simulink model "Adaptive controller"  (R2023b)
settings: Solver=VariableStepAuto  StartTime=0.0  StopTime=100  RelTol=1e-3
InitFcn:
  | clear
  | 
  | % % ---prof params---
  | % b0= 20;
  | % a1= 9;
  | % a0= 20;
  | %
  | % am1= 5;
  | % am0= 6;
  | 
  | % % ---My params ---
  | b0= 3;
  | a1= 3; % previously 3
  | a0= -1; % previously 1
  | 
  | am1= 2;
  | am0= 1;
  | 
  | b0_bar=0.01;
  | gamma0=3000;
  | lambda=1;
  | 
  | d1 = 1;
  | d2 = 3;
  | d3 = 5;
  | 
  | umin=0;
  | umax=2;
settings Model: Creator=Admin  LastModifiedBy=Admin

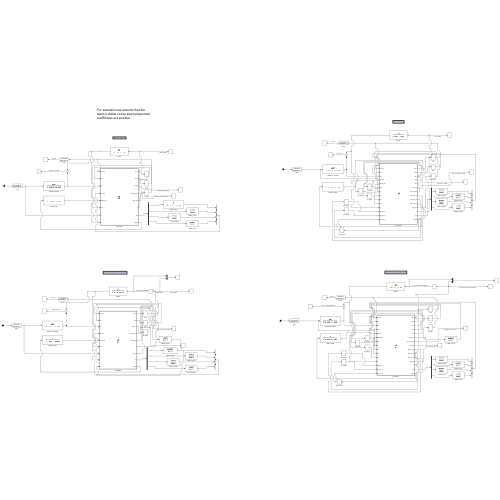
[thumbnail: Simulink's stored preview of the top-level diagram]
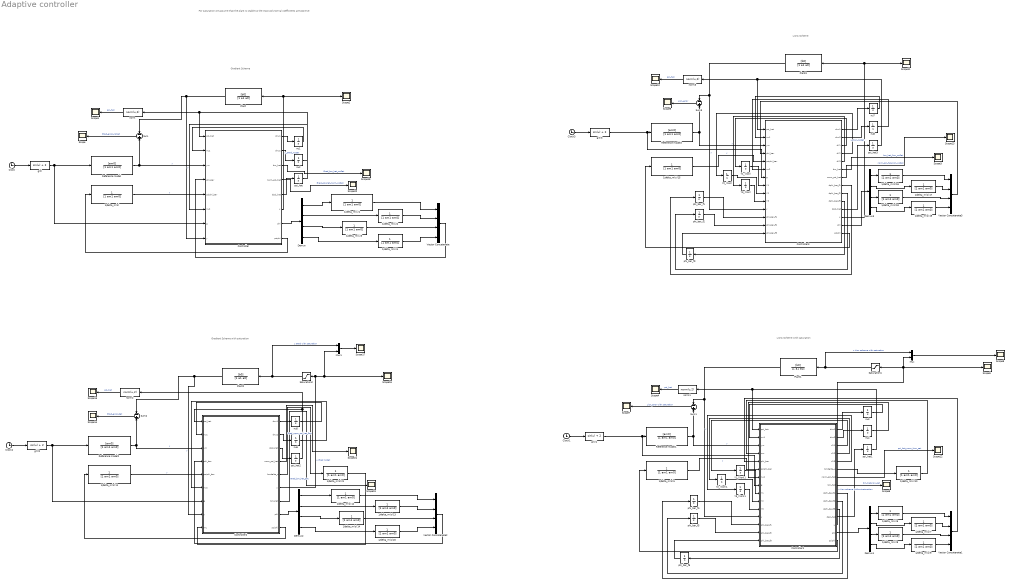
== system Adaptive controller ==
  note: For saturation we assume that the plant is stable so the input polynomial coefficients are positive
  note: Gradient Scheme
  note: Lions Scheme
  note: Lions Scheme with saturation
  note: Gradient Scheme with saturation
  1/delta_m(s){,1..21} (22 alike) : TransferFcn  Denominator=[1 am1 am0]  ParameterTunability=Optimized
  Clock{,1..3} (4 alike) : Clock
  Controller : MATLAB Function  TreatAsAtomicUnit=on
  Controller1 : MATLAB Function  TreatAsAtomicUnit=on
  Controller2 : MATLAB Function  TreatAsAtomicUnit=on
  Controller3 : MATLAB Function  TreatAsAtomicUnit=on
  Demux{,1..3} (4 alike) : Demux
  Mux : Mux  Inputs=2
  Mux1 : Mux  Inputs=2
  Plant{,1..3} (4 alike) : TransferFcn  Numerator=[b0]  Denominator=[1 a1 a0]
  Reference model{,1..3} (4 alike) : TransferFcn  Numerator=[am0]  Denominator=[1 am1 am0]  ParameterTunability=Optimized
  Saturation1 : Saturate  UpperLimit=umax  LowerLimit=umin
  Saturation2 : Saturate  UpperLimit=umax  LowerLimit=umin
  Scope{,1..21} (22 alike) : Scope
  Sum{,1..3} (4 alike) : Sum  Inputs=-+
  Vector Concatenate{,1..3} (4 alike) : Concatenate  NumInputs=4
  Y1_(lion) : Integrator  InitialCondition=[0]
  Y1_(lion)1 : Integrator  InitialCondition=[0]
  Y2_(lion) : Integrator  InitialCondition=[0]
  Y2_(lion)1 : Integrator  InitialCondition=[0]
  Y3_(lion) : Integrator  InitialCondition=[0]
  Y3_(lion)1 : Integrator  InitialCondition=[0]
  g(t){,1..3} (4 alike) : MATLABFcn  MATLABFcn=sin(u) + 2
  norm{,1..3} (4 alike) : MATLABFcn  MATLABFcn=norm(u,2)
  nu{1..8} (8 alike) : Integrator
  phi_bar_f{1..6} (6 alike) : Integrator  InitialCondition=zeros(4,1)
  psi_hat{,1..3} (4 alike) : Integrator  InitialCondition=[0;0;0;1]
  wires:
  1/delta_m(s)1/1 -> Vector Concatenate/1
  Demux/4 -> 1/delta_m(s)4/1
  Demux/1 -> 1/delta_m(s)1/1
  1/delta_m(s)3/1 -> Vector Concatenate/3
  Controller/6(u) -> Scope2/1, Plant/1  "u_Grad_noSat"
  Controller/8(psiphi) -> 1/delta_m(s)/1
  1/delta_m(s)/1 -> Controller/5(psiphi_bar)  "y"
  Plant/1 -> Controller/8(y), Sum/1  "y"
  Controller/2(dnu2) -> nu2/1
  Clock/1 -> g(t)/1
  g(t)/1 -> Controller/7(g), Reference model/1
  Controller/7(phi) -> Demux/1
  Demux/2 -> 1/delta_m(s)2/1
  Reference model/1 -> Controller/3(ym), Sum/2  "y"
  nu1/1 -> Controller/2(nu1)
  Controller/5(dpsi_hat) -> psi_hat/1
  nu2/1 -> Controller/6(nu2)
  psi_hat/1 -> norm/1, Controller/1(psi_hat)
  1/delta_m(s)4/1 -> Vector Concatenate/4
  norm/1 -> Scope1/1  "psi_hat"
  Controller/1(dnu1) -> nu1/1
  Sum/1 -> Scope/1  "Grad_error_noSat"
  Vector Concatenate/1 -> Controller/4(phi_bar)
  Demux/3 -> 1/delta_m(s)3/1
  1/delta_m(s)2/1 -> Vector Concatenate/2
  norm3/1 -> Scope10/1  "psi_hat"
  Vector Concatenate3/1 -> Controller3/4(phi_bar)
  1/delta_m(s)19/1 -> Vector Concatenate3/4
  g(t)3/1 -> Controller3/7(g), Reference model3/1
  1/delta_m(s)17/1 -> Vector Concatenate3/2
  Controller3/12(u) -> Plant3/1, Scope11/1  "u_lion_noSat"
  nu7/1 -> Controller3/2(nu1)
  Controller3/8(dphi_bar_f1) -> phi_bar_f1/1
  Controller3/9(dphi_bar_f2) -> phi_bar_f2/1
  Sum3/1 -> Scope9/1  "Lion_error"
  Demux3/4 -> 1/delta_m(s)19/1
  phi_bar_f3/1 -> Controller3/14(phi_bar_f3)
  1/delta_m(s)18/1 -> Vector Concatenate3/3
  nu8/1 -> Controller3/6(nu2)
  Reference model3/1 -> Sum3/2, Controller3/3(ym)  "y"
  1/delta_m(s)15/1 -> Controller3/5(psiphi_bar)  "y"
  phi_bar_f2/1 -> Controller3/13(phi_bar_f2)
  Y1_(lion)/1 -> Controller3/8(Y1)
  Demux3/2 -> 1/delta_m(s)17/1
  phi_bar_f1/1 -> Controller3/12(phi_bar_f1)
  Controller3/3(dY1) -> Y1_(lion)/1
  Plant3/1 -> Controller3/11(y), Sum3/1  "y"
  Controller3/4(dY2) -> Y2_(lion)/1
  psi_hat3/1 -> Controller3/1(psi_hat), norm3/1
  Y3_(lion)/1 -> Controller3/10(Y3)
  Controller3/5(dY3) -> Y3_(lion)/1
  Demux3/1 -> 1/delta_m(s)16/1
  Y2_(lion)/1 -> Controller3/9(Y2)
  Controller3/1(dnu1) -> nu7/1
  Demux3/3 -> 1/delta_m(s)18/1
  Controller3/10(dphi_bar_f3) -> phi_bar_f3/1
  Clock3/1 -> g(t)3/1
  Controller3/11(dpsi_hat) -> psi_hat3/1
  Controller3/14(psiphi) -> 1/delta_m(s)15/1
  1/delta_m(s)16/1 -> Vector Concatenate3/1
  Controller3/13(phi) -> Demux3/1
  Controller3/2(dnu2) -> nu8/1
  Controller3/6(bm_hat) -> Scope3/1  "bm_hat_lion_noSat"
  Saturation1/1 -> Mux/1, Plant1/1  "u Lion scheme with saturation"
  Controller1/8(bm_hat) -> Scope6/1  "bm_hat_lion_sat"
  phi_bar_f4/1 -> Controller1/13(phi_bar_f1)
  Plant1/1 -> Controller1/12(y), Sum1/1  "y"
  Controller1/1(dnu1) -> nu3/1
  Controller1/14(phi) -> Demux1/1
  norm1/1 -> Scope4/1  "psi_hat"
  Controller1/15(psiphi) -> 1/delta_m(s)5/1
  Demux1/4 -> 1/delta_m(s)9/1
  Controller1/2(dnu2) -> nu4/1
  1/delta_m(s)6/1 -> Vector Concatenate1/1
  Controller1/11(dphi_bar_f3) -> phi_bar_f6/1
  Controller1/5(dY3) -> Y3_(lion)1/1
  Clock1/1 -> g(t)1/1
  Demux1/2 -> 1/delta_m(s)7/1
  nu3/1 -> Controller1/2(nu1)
  Reference model1/1 -> Sum1/2, Controller1/3(ym)  "y"
  Controller1/3(dY1) -> Y1_(lion)1/1
  1/delta_m(s)5/1 -> Controller1/6(psiphi_bar)  "y"
  Demux1/1 -> 1/delta_m(s)6/1
  Controller1/13(u) -> Scope5/1, Saturation1/1, Mux/2  "u Lion scheme without saturation"
  Y3_(lion)1/1 -> Controller1/11(Y3)
  Y1_(lion)1/1 -> Controller1/9(Y1)
  Demux1/3 -> 1/delta_m(s)8/1
  Controller1/4(dY2) -> Y2_(lion)1/1
  Controller1/9(dphi_bar_f1) -> phi_bar_f4/1
  nu4/1 -> Controller1/7(nu2)
  1/delta_m(s)9/1 -> Vector Concatenate1/4
  psi_hat1/1 -> Controller1/1(psi_hat), norm1/1
  phi_bar_f5/1 -> Controller1/14(phi_bar_f2)
  phi_bar_f6/1 -> Controller1/15(phi_bar_f3)
  1/delta_m(s)8/1 -> Vector Concatenate1/3
  Sum1/1 -> Scope7/1  "Lion_error with saturation"
  Vector Concatenate1/1 -> Controller1/5(phi_bar)
  Controller1/10(dphi_bar_f2) -> phi_bar_f5/1
  Y2_(lion)1/1 -> Controller1/10(Y2)
  1/delta_m(s)7/1 -> Vector Concatenate1/2
  Controller1/12(dpsi_hat) -> psi_hat1/1
  g(t)1/1 -> Controller1/8(g), Reference model1/1
  Controller1/6(bmdelta_u) -> 1/delta_m(s)10/1
  1/delta_m(s)10/1 -> Controller1/4(mu)
  Mux/1 -> Scope8/1
  Controller1/7(norm_psi_hat) -> Scope12/1  "psi_hat_norm_Lion_sat"
  Controller3/7(norm_psi_hat) -> Scope13/1  "norm_psi_hat_lion_noSat"
  Demux2/4 -> 1/delta_m(s)20/1
  Demux2/1 -> 1/delta_m(s)12/1
  1/delta_m(s)11/1 -> Controller2/5(psiphi_bar)  "y"
  psi_hat2/1 -> norm2/1, Controller2/1(psi_hat)
  nu6/1 -> Controller2/6(nu2)
  g(t)2/1 -> Controller2/7(g), Reference model2/1
  Controller2/6(u) -> Scope16/1, Mux1/2, Saturation2/1  "u Grad noSat"
  nu5/1 -> Controller2/2(nu1)
  1/delta_m(s)14/1 -> Vector Concatenate2/3
  Clock2/1 -> g(t)2/1
  1/delta_m(s)20/1 -> Vector Concatenate2/4
  Controller2/2(dnu2) -> nu6/1
  Sum2/1 -> Scope14/1  "Grad_error_Sat"
  Demux2/3 -> 1/delta_m(s)14/1
  Vector Concatenate2/1 -> Controller2/4(phi_bar)
  Reference model2/1 -> Sum2/2, Controller2/3(ym)  "y"
  Controller2/8(phi) -> Demux2/1
  1/delta_m(s)13/1 -> Vector Concatenate2/2
  Demux2/2 -> 1/delta_m(s)13/1
  Controller2/1(dnu1) -> nu5/1
  Controller2/3(dpsi_hat) -> psi_hat2/1
  Controller2/9(psiphi) -> 1/delta_m(s)11/1
  Plant2/1 -> Controller2/8(y), Sum2/1  "y"
  norm2/1 -> Scope15/1  "psi_hat"
  1/delta_m(s)12/1 -> Vector Concatenate2/1
  Saturation2/1 -> Mux1/1, Plant2/1  "u Grad with saturation"
  Mux1/1 -> Scope17/1
  Controller/3(bm_hat) -> Scope18/1  "Grad_bm_hat_noSat"
  Controller2/7(bm_hat) -> Scope19/1  "Grad_bm_hat_Sat"
  Controller/4(norm_psi_hat) -> Scope20/1  "Grad_psi_hat_norm_noSat"
  Controller2/4(norm_psi_hat) -> Scope21/1  "Grad_norm_psi_hat_Sat"
  Controller2/5(bmdelta_u) -> 1/delta_m(s)21/1
  1/delta_m(s)21/1 -> Controller2/9(mu)

== matlab function Adaptive controller/Controller2 ==
  data: psi_hat input; dnu1 output; nu1 input; ym input; phi_bar input; psiphi_bar input; nu2 input; g input; y input; b0_bar parameter; mu input; dnu2 output; dpsi_hat output; norm_psi_hat output; bmdelta_u output; u output; bm_hat output; phi output; psiphi output; gamma0 parameter; am0 parameter; lambda parameter; umin parameter; umax parameter
function [dnu1, dnu2, dpsi_hat, norm_psi_hat, bmdelta_u, u, bm_hat, phi, psiphi] = fcn(psi_hat, nu1, ym, phi_bar,....
    psiphi_bar, nu2, g, y, b0_bar, mu, gamma0, am0, lambda, umin, umax)


% === Initialize Outputs ===
dnu1 = 0;
dnu2 = 0;
dpsi_hat = zeros(4,1);
u = 0;
psi_hat = psi_hat(:);  
phi_bar = phi_bar(:);
phi = zeros(4,1);
psiphi = 0;
bmdelta_u = 0;

% Extract parameters as COLUMN vector
theta_hat = psi_hat(1:3);   

bm_hat = psi_hat(4);        

% Regressor
omega = [y; nu1; nu2];     

% Tracking error
epsilon = ym - y - mu;

% Augmented error
epsilon_hat = epsilon - (psi_hat' * phi_bar) + psiphi_bar;

% Control law — now dimensionally correct
u = (1 / bm_hat) * (-theta_hat' * omega + am0 * g);

% === Apply Saturation ===
Us = u;
if u <= umin
    Us = umin;
elseif u >= umax
    Us = umax;
end

% === Correction Term ===
bmdelta_u = bm_hat * (u - Us);
 
phi = [-omega; -Us];
psiphi = psi_hat'*phi;
omega_bar = -[phi_bar(1); phi_bar(2); phi_bar(3)];

gamma0=gamma0*eye(4); coord=[0;0;0;1];
 
if bm_hat<b0_bar
    gamma0=gamma0*(eye(4)-coord*coord');
end
 
% Normalize gamma based on regressor energy
denom = 1 + omega_bar' * omega_bar;  
gamma = gamma0 / denom;       

% Final adaptation law
dpsi_hat = gamma * phi_bar * epsilon_hat;

% Derivatives for filters
dnu1 = -lambda*nu1+y;
dnu2 = -lambda*nu2+Us;

% Output psiphi if needed
psiphi = psi_hat' * phi;

% Compute Euclidean norm of psi_hat
norm_psi_hat = norm(psi_hat);  
 
end

== matlab function Adaptive controller/Controller3 ==
  data: psi_hat input; dnu1 output; nu1 input; ym input; phi_bar input; psiphi_bar input; nu2 input; g input; Y1 input; Y2 input; Y3 input; y input; dnu2 output; dY1 output; dY2 output; dY3 output; bm_hat output; norm_psi_hat output; dphi_bar_f1 output; dphi_bar_f2 output; dphi_bar_f3 output; dpsi_hat output; u output; phi output; psiphi output; b0_bar parameter; phi_bar_f1 input; phi_bar_f2 input; phi_bar_f3 input; gamma0 parameter; am0 parameter; lambda parameter; d1 parameter; d2 parameter; d3 parameter
function [dnu1, dnu2, dY1, dY2, dY3,bm_hat, norm_psi_hat, dphi_bar_f1, dphi_bar_f2, dphi_bar_f3, dpsi_hat, u, phi, psiphi] = ...
    fcn(psi_hat, nu1, ym, phi_bar, psiphi_bar, nu2, g, Y1, Y2, Y3, y, b0_bar, ...
        phi_bar_f1, phi_bar_f2, phi_bar_f3, gamma0, am0, lambda, d1, d2, d3)

% === Initialize Outputs ===
dnu1 = 0;
dnu2 = 0;
dY1 = 0;
dY2 = 0;
dY3 = 0;
dphi_bar_f1 = zeros(4,1);
dphi_bar_f2 = zeros(4,1);
dphi_bar_f3 = zeros(4,1);
dpsi_hat = zeros(4,1);
u = 0;
phi = zeros(4,1);
psiphi = 0;

% === Input Handling ===
psi_hat = psi_hat(:);           
phi_bar = phi_bar(:);           
psiphi_bar = psiphi_bar(:);

% Filter states
phi_bar_f1 = phi_bar_f1(:);     
phi_bar_f2 = phi_bar_f2(:);     
phi_bar_f3 = phi_bar_f3(:);     

% === Extract Parameters ===
theta_hat = psi_hat(1:3);       
bm_hat = psi_hat(4);            

% === Regressor ===
omega = [y; nu1; nu2];          

% === Tracking Error ===
epsilon = ym - y;              

% === Augmented Error Estimate ===
y_hat = epsilon + psiphi_bar;   

% === Control Law ===
u = (1 / bm_hat) * (-theta_hat' * omega + am0 * g);

% === Extended Regressor ===
phi = [-omega; -u];             
psiphi = psi_hat' * phi;        

% === Adaptation Gain Normalization ===
omega_bar = -[phi_bar(1); phi_bar(2); phi_bar(3)]; 
denom = 1 + omega_bar' * omega_bar;  
gamma_scalar = gamma0 / denom;
gamma = gamma_scalar * eye(4);       

% === Derivatives of Filtered Signals ===
dY1 = -d1*Y1 + d1*y_hat;
dY2 = -d2*Y2 + d2*y_hat;
dY3 = -d3*Y3 + d3*y_hat;

dphi_bar_f1 = -d1*phi_bar_f1 + d1*phi_bar;
dphi_bar_f2 = -d2*phi_bar_f2 + d2*phi_bar;
dphi_bar_f3 = -d3*phi_bar_f3 + d3*phi_bar;

% === Compute Parametric Error for Each Filter Channel ===
E1 = Y1 - phi_bar_f1' * psi_hat;  
E2 = Y2 - phi_bar_f2' * psi_hat;  
E3 = Y3 - phi_bar_f3' * psi_hat;  

% === Final Adaptation Law ===
TotalUpdate = phi_bar_f1 * E1 + phi_bar_f2 * E2 + phi_bar_f3 * E3;
dpsi_hat = gamma * TotalUpdate;  

% === State Filters Derivatives ===
dnu1 = -lambda * nu1 + y;
dnu2 = -lambda * nu2 + u;

% Compute Euclidean norm of psi_hat
norm_psi_hat = norm(psi_hat);  

% === Output psiphi ===
psiphi = psi_hat' * phi;

end

== matlab function Adaptive controller/Controller1 ==
  data: psi_hat input; dnu1 output; nu1 input; ym input; mu input; phi_bar input; psiphi_bar input; nu2 input; g input; Y1 input; Y2 input; Y3 input; y input; dnu2 output; dY1 output; dY2 output; dY3 output; bmdelta_u output; norm_psi_hat output; bm_hat output; dphi_bar_f1 output; dphi_bar_f2 output; dphi_bar_f3 output; dpsi_hat output; u output; phi output; psiphi output; b0_bar parameter; phi_bar_f1 input; phi_bar_f2 input; phi_bar_f3 input; gamma0 parameter; am0 parameter; lambda parameter; d1 parameter; d2 parameter; d3 parameter; umin parameter; umax parameter
function [dnu1, dnu2, dY1, dY2, dY3, bmdelta_u, norm_psi_hat, bm_hat, dphi_bar_f1, dphi_bar_f2, dphi_bar_f3, dpsi_hat, u, phi, psiphi] = ...
    fcn(psi_hat, nu1, ym, mu, phi_bar, psiphi_bar, nu2, g, Y1, Y2, Y3, y, b0_bar, ...
        phi_bar_f1, phi_bar_f2, phi_bar_f3, gamma0, am0, lambda, d1, d2, d3, umin, umax)

% === Initialize Outputs ===
dnu1 = 0;
dnu2 = 0;
dY1 = 0;
dY2 = 0;
dY3 = 0;
dphi_bar_f1 = zeros(4,1);
dphi_bar_f2 = zeros(4,1);
dphi_bar_f3 = zeros(4,1);
dpsi_hat = zeros(4,1);
u = 0;
phi = zeros(4,1);
psiphi = 0;

% === Input Handling ===
psi_hat = psi_hat(:);           
phi_bar = phi_bar(:);           
psiphi_bar = psiphi_bar(:);

% Filter states
phi_bar_f1 = phi_bar_f1(:);     
phi_bar_f2 = phi_bar_f2(:);     
phi_bar_f3 = phi_bar_f3(:);     

% === Extract Parameters ===
theta_hat = psi_hat(1:3);       
bm_hat = psi_hat(4);            

% === Regressor ===
omega = [y; nu1; nu2];          

% === Tracking Error ===
epsilon = ym - y - mu;               

% === Augmented Error Estimate ===
y_hat = epsilon + psiphi_bar;   

% === Control Law ===
u = (1 / bm_hat) * (-theta_hat' * omega + am0 * g);

Us=u;
if u<=umin
    Us=umin;
elseif u>=umax
    Us=umax;
end

bmdelta_u = bm_hat*(u-Us);

% === Extended Regressor ===
phi = [-omega; -Us];             
psiphi = psi_hat' * phi;        

% === Adaptation Gain Normalization ===
omega_bar = -[phi_bar(1); phi_bar(2); phi_bar(3)];  
denom = 1 + omega_bar' * omega_bar;  
gamma_scalar = gamma0 / denom;
gamma = gamma_scalar * eye(4);       

% === Derivatives of Filtered Signals ===
dY1 = -d1*Y1 + d1*y_hat;
dY2 = -d2*Y2 + d2*y_hat;
dY3 = -d3*Y3 + d3*y_hat;

dphi_bar_f1 = -d1*phi_bar_f1 + d1*phi_bar;
dphi_bar_f2 = -d2*phi_bar_f2 + d2*phi_bar;
dphi_bar_f3 = -d3*phi_bar_f3 + d3*phi_bar;

% === Compute Parametric Error for Each Filter Channel ===
E1 = Y1 - phi_bar_f1' * psi_hat;  
E2 = Y2 - phi_bar_f2' * psi_hat;  
E3 = Y3 - phi_bar_f3' * psi_hat;  

% === Final Adaptation Law ===
TotalUpdate = phi_bar_f1 * E1 + phi_bar_f2 * E2 + phi_bar_f3 * E3;
dpsi_hat = gamma * TotalUpdate;  

% Compute Euclidean norm of psi_hat
norm_psi_hat = norm(psi_hat);  

% === State Filters Derivatives ===
dnu1 = -lambda * nu1 + y;
dnu2 = -lambda * nu2 + Us;

% === Output psiphi ===
psiphi = psi_hat' * phi;

end

== matlab function Adaptive controller/Controller ==
  data: psi_hat input; dnu1 output; nu1 input; ym input; phi_bar input; psiphi_bar input; nu2 input; g input; y input; dnu2 output; bm_hat output; norm_psi_hat output; dpsi_hat output; u output; phi output; psiphi output; b0_bar parameter; gamma0 parameter; am0 parameter; lambda parameter
function [dnu1, dnu2, bm_hat, norm_psi_hat, dpsi_hat, u, phi, psiphi] = fcn(psi_hat, nu1, ym, phi_bar, ...
    psiphi_bar, nu2, g, y, b0_bar, gamma0, am0, lambda)


psi_hat = psi_hat(:);     
phi_bar = phi_bar(:);     
psiphi_bar = psiphi_bar(:);

% Extract parameters
theta_hat = psi_hat(1:3); 
bm_hat = psi_hat(4);      

% Regressor
omega = [y; nu1; nu2];    

% Tracking error
epsilon = ym - y;         % Scalar

% Augmented error:̂
epsilon_hat = epsilon - (psi_hat' * phi_bar) + psiphi_bar;

% Control law
u = (1 / bm_hat) * (-theta_hat' * omega + am0 * g);

% Extended regressor
phi = [-omega; -u];      
psiphi = psi_hat' * phi;  

% For adaptation gain conditioning
omega_bar = -[phi_bar(1); phi_bar(2); phi_bar(3)];  

% Adaptation gain gamma0 
gamma0 = gamma0 * eye(4);
coord = [0; 0; 0; 1];

% Projection-like modification if bm_hat < b0_bar
if bm_hat < b0_bar
    gamma0 = gamma0 * (eye(4) - coord*coord');
end

% Normalize gamma based on regressor energy
denom = 1 + omega_bar' * omega_bar;  % Should be scalar
gamma = gamma0 / denom;       

% Final adaptation law
dpsi_hat = gamma * phi_bar * epsilon_hat;

% Derivatives for filters
dnu1 = -lambda * nu1 + y;
dnu2 = -lambda * nu2 + u;

% Output psiphi if needed
psiphi = psi_hat' * phi;

% Compute Euclidean norm of psi_hat
norm_psi_hat = norm(psi_hat);  

end
